simulink model "dorteee"  (R2021b)
settings: Solver=VariableStepAuto  StartTime=0.0  StopTime=0.001  RelTol=1e-3
libraries: spsCurrentMeasurementLib x4, spsVoltageMeasurementLib x4, simulink x3, spsParallelRLCBranchLib x3, spsDCVoltageSourceLib x1, spsDiodeLib x1, spsIdealSwitchLib x1, spspowerguiLib x1
settings Model: Creator=irem3  LastModifiedBy=irem3

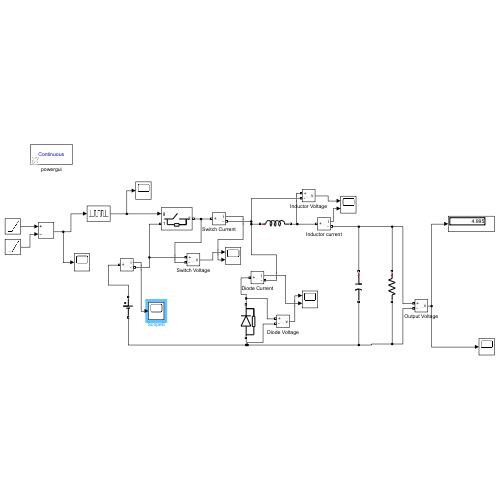
[thumbnail: Simulink's stored preview of the top-level diagram]
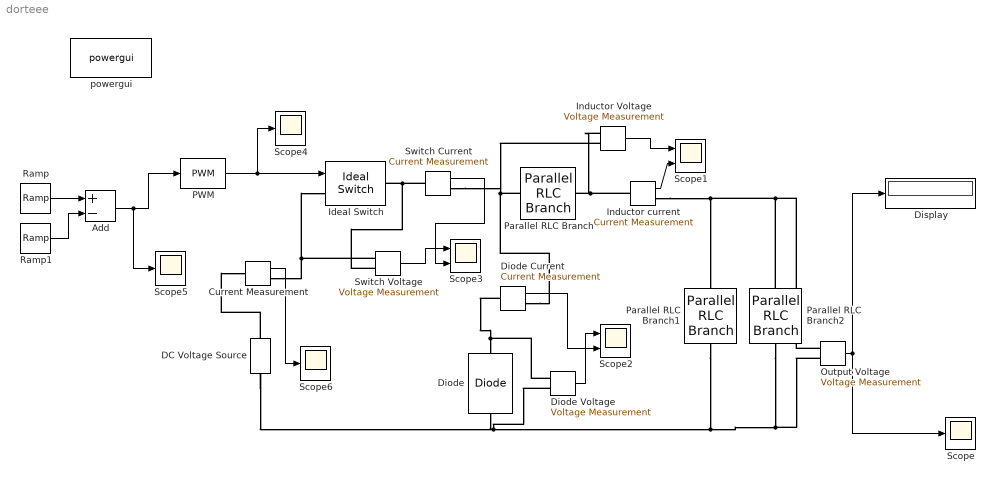
== system dorteee ==
  Add : Sum  Inputs=+-
  Current Measurement : spsCurrentMeasurementLib/Current Measurement  PhasorSimulation=off  OutputType=Complex  PSBequivalent=0
  DC Voltage Source : spsDCVoltageSourceLib/DC Voltage Source  Amplitude=12  Measurements=None
  Diode : spsDiodeLib/Diode  Ron=1e-9  Lon=0  Vf=0.001  IC=0  UseSnubber=0  Rs=500  Cs=250e-9  Measurements=off
  Diode Current : spsCurrentMeasurementLib/Current Measurement  PhasorSimulation=off  OutputType=Complex  PSBequivalent=0
  Diode Voltage : spsVoltageMeasurementLib/Voltage Measurement  PhasorSimulation=off  OutputType=Complex  PSBequivalent=0
  Display : Display
  Ideal Switch : spsIdealSwitchLib/Ideal Switch  Ron=1e-9  Lon=0  IC=0  Rs=1e5  Cs=inf  Measurements=off
  Inductor Voltage : spsVoltageMeasurementLib/Voltage Measurement  PhasorSimulation=off  OutputType=Complex  PSBequivalent=0
  Inductor current : spsCurrentMeasurementLib/Current Measurement  PhasorSimulation=off  OutputType=Complex  PSBequivalent=0
  Output Voltage : spsVoltageMeasurementLib/Voltage Measurement  PhasorSimulation=off  OutputType=Complex  PSBequivalent=0
  PWM : simulink/Discontinuities/PWM  DisableCoverage=on  Period=1/500000  DisallowZeroDutyCycle=off  RunAtFixedTimeIntervals=off  SampleTime=0.1
  Parallel RLC Branch : spsParallelRLCBranchLib/Parallel RLC Branch  LConnTagsString=a  RConnTagsString=__new0  BranchType=L  Resistance=0  Inductance=5e-6  SetiL0=off  InitialCurrent=0  Capacitance=0  Setx0=off  InitialVoltage=0  Measurements=None
  Parallel RLC Branch1 : spsParallelRLCBranchLib/Parallel RLC Branch  LConnTagsString=a  RConnTagsString=__new0  BranchType=C  Resistance=0  Inductance=1e-3  SetiL0=off  InitialCurrent=0  Capacitance=10e-6  Setx0=off  InitialVoltage=0  Measurements=None
  Parallel RLC Branch2 : spsParallelRLCBranchLib/Parallel RLC Branch  LConnTagsString=a  RConnTagsString=__new0  BranchType=R  Resistance=25  Inductance=1e-3  SetiL0=off  InitialCurrent=0  Capacitance=10e-6  Setx0=off  InitialVoltage=0  Measurements=None
  Ramp : simulink/Sources/Ramp  slope=2440  start=0  InitialOutput=0
  Ramp1 : simulink/Sources/Ramp  slope=2440  start=1e-4  InitialOutput=0
  Scope{,4..6} (4 alike) : Scope
  Scope1 : Scope  NumInputPorts=2
  Scope2 : Scope  NumInputPorts=2
  Scope3 : Scope  NumInputPorts=2
  Switch Current : spsCurrentMeasurementLib/Current Measurement  PhasorSimulation=off  OutputType=Complex  PSBequivalent=0
  Switch Voltage : spsVoltageMeasurementLib/Voltage Measurement  PhasorSimulation=off  OutputType=Complex  PSBequivalent=0
  powergui : spspowerguiLib/powergui  Priority=1  SimulationMode=Continuous  SampleTime=50e-6  frequency=60  Iterations=50  frequencyindice=0  Pbase=100e6  ErrMax=1e-4  UnitsV=kV  UnitsW=MW  buscounter=0  FunctionMessages=off  echomessages=off  EnableUseOfTLC=off  CurrentSourceSwitches=off  DisableSnubberDevices=off  DisableRonSwitches=off  DisableVfSwitches=off  DisplayEquations=off  AutomaticDiscreteSolvers=off  SolverType=Tustin/Backward Euler (TBE)  Interpol=off  ExternalGateDelay=off  methode=off  Ts=100  x0status=blocks  SPID=on  SwTol=0  HookPort=off  NonlinearTolerance=1e-4  nMaxIteration=100  ContinueOnMaxIteration=off  RestoreLinks=warning  ResistiveCurrentMeasurement=off  Frange=[0:2:500]  Ylog=off  Xlog=on  ShowGrid=off  save=off  variable=ZData  structure=0  ZoomFFT=off  StartTime=0.0  cycles=1  DisplayStyle=1  fundamental=60  FreqAxis=off  MaxFrequency=1000  frequencyindicesteady=1  RmsSteady=1  display=off
  wires:
  Output Voltage/1 -> Display/1, Scope/1
  PWM/1 -> Scope4/1, Ideal Switch/1
  Inductor Voltage/1 -> Scope1/1
  Inductor current/1 -> Scope1/2
  Diode Voltage/1 -> Scope2/1
  Diode Current/1 -> Scope2/2
  Switch Voltage/1 -> Scope3/1
  Switch Current/1 -> Scope3/2
  Ramp/1 -> Add/1
  Ramp1/1 -> Add/2
  Add/1 -> Scope5/1, PWM/1
  Current Measurement/1 -> Scope6/1
  connections:
  Switch Voltage/LConn1 -- Ideal Switch/LConn1 -- Current Measurement/RConn1
  Parallel RLC Branch/LConn1 -- Switch Current/RConn1 -- Inductor Voltage/LConn2 -- Diode Current/RConn1
  Parallel RLC Branch1/RConn1 -- Diode Voltage/LConn2 -- Diode/LConn1 -- DC Voltage Source/LConn1 -- Parallel RLC Branch2/RConn1 -- Output Voltage/LConn2
  Output Voltage/LConn1 -- Parallel RLC Branch1/LConn1 -- Inductor current/RConn1 -- Parallel RLC Branch2/LConn1
  Inductor current/LConn1 -- Inductor Voltage/LConn1 -- Parallel RLC Branch/RConn1
  Diode Current/LConn1 -- Diode Voltage/LConn1 -- Diode/RConn1
  Switch Current/LConn1 -- Switch Voltage/LConn2 -- Ideal Switch/RConn1
  DC Voltage Source/RConn1 -- Current Measurement/LConn1
